simulink model "Vehicle_Model_999_Modular"  (R2025b)
settings: Solver=ode23tb  StartTime=0.0  StopTime=20  MaxStep=0.001  RelTol=1e-3
values from neighbouring files (symbols this model uses):
  aero_par = struct()    [Load_aero_parameters.m]
  init_r = 0    [Run_this_first.m]
  init_vx = 0    [Run_this_first.m]
  init_vy = 0    [Run_this_first.m]
  m = Par.m    [LapSim_Endurance_final_ts_v2.m]    (also in Lap_Sim_Final_inverse.m = Par.Mass; Lapsim_Endurance_final_ts.m; New_LapSim_final_ts_v1.m = Par.Mass; Torque_vectoring_lookup_table_v3.m = 270)
  Par = struct()    [Load_vehicle_parameters.m]
  sus_par = struct()    [Load_sus_parameters.m]
  TireData = []    [Lapsim_final_for_app.m]
  V_ref = 45    [Run_this_first.m]
undefined symbols (not defined in the file or in its folder): Battery, Brake_Val, HP, Ki_data, Kp_data, Motor, steer_input, Steer_Val, Throttle_Val, vx_breakpoints
libraries: simulink x7, autolibshared x2, BatteryEstimators x1, simulink_extras x1
(part 3 of 3)

== matlab function Vehicle_Model_999_Modular/Drivetrain/Thermal/MATLAB Function ==
  settings: updateMethod=DISCRETE  sampleTime=1
  data: Q_total output size=1; I_rms input; Speed_RPM input; P_iron_rotor input; T_motor_K input; T_motor_C output; R_actual output; kt_actual output
function [Q_total, T_motor_C, R_actual, kt_actual] = motor_thermal_logic(I_rms, Speed_RPM, P_iron_rotor, T_motor_K)
    %#codegen
    
    %% 1. Force outputs to be SCALAR doubles
    % This stops the "variable-size matrix" error
    Q_total   = double(0); 
    T_motor_C = double(0);
    R_actual  = double(0);
    kt_actual = double(0);

    %% 2. Constants from Fischer Datasheet
    R_ref   = 0.126;    % Phase resistance at 20°C
    kt_ref  = 0.492;    % Torque constant
    alpha   = 0.00393;  % Temp coefficient for Copper
    gamma_m = 0.001;    % Magnet flux fade (0.1% per degC)
    
    %% 3. Unit Conversion & Calculations
    T_kelvin = double(T_motor_K(1));
    T_motor_C = T_motor_K - 273.15; % Kelvin to Celsius
    
    % Ensure T_motor_C doesn't cause math errors if feedback is zero at start
    R_actual = R_ref * (1 + alpha * (T_motor_C - 20)); 
    kt_actual = kt_ref * (1 - gamma_m * (T_motor_C - 20)); 
    
    % Force I_rms to be treated as a single scalar value
    I_val = double(I_rms(1));
    P_cu = 3 * (I_val^2) * R_actual; 
    
    % Final sum forced to scalar double
    Q_total = P_cu + double(P_iron_rotor(1)); 
end

== matlab function Vehicle_Model_999_Modular/E-powertrain/Motor/Motor with Field Weakening ==
  data: kt input; rpm_4x1 input; Torque_Nm_vec output; throttle_scalar input; v_dc_bus input; Motor parameter; I_dc_total output size=[1]; P_total_sum output size=[1]
function [Torque_Nm_vec, I_dc_total,P_total_sum] = fcn(kt, rpm_4x1, throttle_scalar, v_dc_bus, Motor)
    % Inputs:
    %   rpm_4x1         : [FL; FR; RL; RR] wheel speeds in RPM
    %   throttle_scalar : Driver input (0 to 1)
    %   v_dc_bus        : Battery voltage (V)
    %   Motor           : Struct containing constants
    
    % --- 1. Distribute Inputs ---
    % We apply the same throttle to both motors for now.
    % We extract the Rear-Left (index 3) and Rear-Right (index 4) speeds.
    rpm_targets = [rpm_4x1(3); rpm_4x1(4)]; 
    throttle_vec = [throttle_scalar; throttle_scalar];
    psi_m = kt / (1.5 * Motor.p * sqrt(2)); 

    % Initialize storage
    Torque_Nm_vec = zeros(2, 1); % [T_RL; T_RR]
    P_elec_vec = zeros(2, 1);
    
    for i = 1:2
        % --- 2. Redline & Mechanical Limit Check ---
        if abs(rpm_targets(i)) >= Motor.n_max
            continue; % Torque and Power remain 0
        end

        % --- 3. Electrical Conversions ---
        omega_m = rpm_targets(i) * (2*pi/60);
        omega_e = max(abs(omega_m * Motor.p), 0.1); 
        V_max_phase = v_dc_bus / sqrt(3);
        I_cmd_peak = Motor.I_max_rms * sqrt(2) * throttle_vec(i);

        % --- 4. Region Selection: MTPA vs Field Weakening ---
        V_req_mtpa = omega_e * sqrt((Motor.L * I_cmd_peak)^2 + psi_m^2);
        
        if V_req_mtpa <= V_max_phase
            id = 0;
            iq = I_cmd_peak;
        else
            % Field Weakening logic for Fischer Motor
            a = Motor.L^2;
            b = 2 * Motor.L * psi_m;
            c = Motor.psi_m^2 + (Motor.L * I_cmd_peak)^2 - (V_max_phase / omega_e)^2;
            
            id = (-b + sqrt(max(0, b^2 - 4 * a * c))) / (2 * a);
            id = max(min(id, 0), -I_cmd_peak); 
            iq = sqrt(max(0, I_cmd_peak^2 - id^2));
        end

        % --- 5. Torque and Power Calculation ---
        T_gen = 1.5 * Motor.p * psi_m * iq;
        Torque_Nm_vec(i) = min(T_gen, Motor.T_peak_limit);

        % P_elec = P_mechanical + P_copper_losses
        P_mech = abs(Torque_Nm_vec(i) * omega_m);
        P_copper = 3 * 0.126 * (I_cmd_peak / sqrt(2))^2;
        P_elec_vec(i) = P_mech + P_copper;
    end

    % --- 6. Battery Summation ---
    P_total_sum = sum(P_elec_vec);
    if v_dc_bus > 20
        % Calculate total current draw for the Molicel P45B pack
        I_dc_total = P_total_sum / (0.95 * v_dc_bus);

    else
        I_dc_total = 0;
    end
end

== matlab function Vehicle_Model_999_Modular/Vehicle dynamics/Fx, Fy calculations/Tyre_relaxation/MATLAB Function ==
  data: Fx_ss input; Fx_dot output; Fx_act input; Vx input
function Fx_dot = fcn(Fx_ss, Fx_act, Vx)
    % Fx_ss: Force from Magic Formula block
    % Fx_act: The current integrated force
    % Vx: Longitudinal velocity
    sigma_x = 0.1;
    % Use a small epsilon to avoid division by zero at standstill
    Vx_mod = max(abs(Vx), 0.05); 
    
    % The differential equation
    Fx_dot = (Vx_mod / sigma_x).* (Fx_ss - Fx_act);
end

== matlab function Vehicle_Model_999_Modular/Vehicle dynamics/Fx, Fy calculations/Visualise_Fy_B/MATLAB Function ==
  data: Fy_tire input; Fy_B_fl output; Fy_B_fr output; Fy_B_rl output; Fy_B_rr output
function [Fy_B_fl,Fy_B_fr,Fy_B_rl,Fy_B_rr]  = fcn(Fy_tire)

Fy_B_fl = Fy_tire(1);

Fy_B_fr = Fy_tire(2);

Fy_B_rl = Fy_tire(3);

Fy_B_rr = Fy_tire(4);

end

== matlab function Vehicle_Model_999_Modular/Drivetrain/MATLAB Function ==
  data: T_fl output; T_fr output
function [T_fl,T_fr] = fcn()

T_fl = 0;
T_fr = 0;

== matlab function Vehicle_Model_999_Modular/Vehicle dynamics/Suspension/Camber/DynamicCamber_FromHP_Zmeters ==
  data: Camber output; Zs input; Zs_static input; sus_par parameter; HP parameter; dynamic_camber_visualisation output; static_camber_visualisation output
function [Camber,dynamic_camber_visualisation,static_camber_visualisation] = DynamicCamber_FromHP_Zmeters(Zs,Zs_static,sus_par, HP)
%#codegen
% z_* : wheel vertical displacement (meters, + = bump)
% HP  : hardpoints (mm)
% Output Camber [4x1] radians (dynamic, zeroed at ride height)

% Use this if you have different camber angles for front and rear wheels.
% static_camber_4x1 = [sus_par.Camber_static_f.*ones(2,1) ; ...
                       ...sus_par.Camber_static_r.*ones(2,1)];   
% Assigning values of Zs                           
Zs_1 = Zs(1);
Zs_2 = Zs(2);
Zs_3 = Zs(3);
Zs_4 = Zs(4);
% Assigning values of Zs                           
Zs_1_static = Zs_static(1);
Zs_2_static = Zs_static(2);
Zs_3_static = Zs_static(3);
Zs_4_static = Zs_static(4);
                  
static_camber_4x1 = sus_par.Camber_static.*ones(4,1);

z_FL_static = Zs_1_static * sus_par.Motion_ratio_f;
z_FR_static = Zs_2_static * sus_par.Motion_ratio_f;
z_RL_static = Zs_3_static * sus_par.Motion_ratio_r;
z_RR_static = Zs_4_static * sus_par.Motion_ratio_r;

z_FL = Zs_1 * sus_par.Motion_ratio_f;
z_FR = Zs_2 * sus_par.Motion_ratio_f;
z_RL = Zs_3 * sus_par.Motion_ratio_r;
z_RR = Zs_4 * sus_par.Motion_ratio_r;

%% Convert meters -> mm   (wheel displacement in mm)
zw_FL = z_FL * 1000;
zw_FR = z_FR * 1000;
zw_RL = z_RL * 1000;
zw_RR = z_RR * 1000;

%% Convert meters -> mm   (wheel displacement in mm for _static calculations)
zw_FL_static = z_FL_static * 1000;
zw_FR_static = z_FR_static * 1000;
zw_RL_static = z_RL_static * 1000;
zw_RR_static = z_RR_static * 1000;

%% Absolute camber from geometry

    Camber_FL_d = solveCorner_camber(zw_FL,...
        HP.Front.UCA_F, HP.Front.UCA_R, HP.Front.UCA_O, ...
        HP.Front.LCA_F, HP.Front.LCA_R, HP.Front.LCA_O, ...
        HP.Front.TCP,  1);
    Camber_FL_s = solveCorner_theta(zw_FL_static,...
        HP.Front.UCA_F, HP.Front.UCA_R, HP.Front.UCA_O, ...
        HP.Front.LCA_F, HP.Front.LCA_R, HP.Front.LCA_O, ...
        HP.Front.TCP,  1);

Camber_FL = -Camber_FL_s + Camber_FL_d;

    Camber_FR_d = solveCorner_camber(zw_FR, ...
        HP.Front.UCA_F, HP.Front.UCA_R, HP.Front.UCA_O, ...
        HP.Front.LCA_F, HP.Front.LCA_R, HP.Front.LCA_O, ...
        HP.Front.TCP, -1);
    Camber_FR_s = solveCorner_theta(zw_FR_static, ...
        HP.Front.UCA_F, HP.Front.UCA_R, HP.Front.UCA_O, ...
        HP.Front.LCA_F, HP.Front.LCA_R, HP.Front.LCA_O, ...
        HP.Front.TCP, -1);

Camber_FR = -Camber_FR_d - Camber_FR_s;

    Camber_RL_d =  solveCorner_camber(zw_RL, ...
        HP.Rear.UCA_F, HP.Rear.UCA_R, HP.Rear.UCA_O, ...
        HP.Rear.LCA_F, HP.Rear.LCA_R, HP.Rear.LCA_O, ...
        HP.Rear.TCP,  1);
    Camber_RL_s = solveCorner_theta(zw_RL_static, ...
        HP.Rear.UCA_F, HP.Rear.UCA_R, HP.Rear.UCA_O, ...
        HP.Rear.LCA_F, HP.Rear.LCA_R, HP.Rear.LCA_O, ...
        HP.Rear.TCP,  1);

Camber_RL = Camber_RL_d - Camber_RL_s;

    Camber_RR_d = solveCorner_camber(zw_RR, ...
        HP.Rear.UCA_F, HP.Rear.UCA_R, HP.Rear.UCA_O, ...
        HP.Rear.LCA_F, HP.Rear.LCA_R, HP.Rear.LCA_O, ...
        HP.Rear.TCP, -1);
    Camber_RR_s = solveCorner_theta(zw_RR_static, ...
        HP.Rear.UCA_F, HP.Rear.UCA_R, HP.Rear.UCA_O, ...
        HP.Rear.LCA_F, HP.Rear.LCA_R, HP.Rear.LCA_O, ...
        HP.Rear.TCP, -1);

Camber_RR = -Camber_RR_d - Camber_RR_s;

Camber_abs = [Camber_FL; Camber_FR; Camber_RL; Camber_RR];

%% Dynamic camber (zeroed at ride height)
Camber = Camber_abs + static_camber_4x1;
dynamic_camber_visualisation = [Camber_FL_d;Camber_FR_d;Camber_RL_d;Camber_RR_d];
static_camber_visualisation = [Camber_FL_s;Camber_FR_s;Camber_RL_s;Camber_RR_s];

end

%% Helper function - 1
function Camber = solveCorner_camber(z,UF,UR,UO,LF,LR,LO,TCP,side)
%#codegen
% Returns camber in radians (negative = negative camber)    
%% Mirror for vehicle side
UF(2)=UF(2)*side; UR(2)=UR(2)*side; UO(2)=UO(2)*side;
LF(2)=LF(2)*side; LR(2)=LR(2)*side; LO(2)=LO(2)*side;
TCP(2)=TCP(2)*side;

%% Apply wheel vertical displacement (mm)
UO(3)=UO(3) + z;
LO(3)=LO(3) + z;
TCP(3)=TCP(3) + z;

%% Inner pivots (front view)
UiY = (UF(2)+UR(2))/2;
UiZ = (UF(3)+UR(3))/2;

LiY = (LF(2)+LR(2))/2;
LiZ = (LF(3)+LR(3))/2;

%% Slopes of upper & lower arms
dYU = (UO(2)-UiY);
dYL = (LO(2)-LiY);

if abs(dYU) < 1e-9, dYU = sign(dYU)*1e-9; end
if abs(dYL) < 1e-9, dYL = sign(dYL)*1e-9; end

mU = (UO(3)-UiZ)/dYU;
mL = (LO(3)-LiZ)/dYL;

cU = UiZ - mU*UiY;
cL = LiZ - mL*LiY;

%% Instant Center
den = (mU-mL);
if abs(den) < 1e-9, den = sign(den)*1e-9; end

ICy = (cL-cU)/den;
ICz = mU*ICy + cU;

%% Camber from IC -> Contact Patch (correct definition)
dY = ICy - TCP(2);     % lateral
dZ = ICz - TCP(3);    % vertical

if abs(dZ) < 1e-9, dZ = sign(dZ)*1e-9; end
Camber = -atan(dY/dZ);
end

%% Helper function - 2
function Theta = solveCorner_theta(Z_static,UF,UR,UO,LF,LR,LO,TCP,side)
%% Mirror for vehicle side
    UF(2)=UF(2)*side; UR(2)=UR(2)*side; UO(2)=UO(2)*side;
    LF(2)=LF(2)*side; LR(2)=LR(2)*side; LO(2)=LO(2)*side;
    TCP(2)=TCP(2)*side;
    
    %% Apply wheel vertical displacement (mm)
    UO(3)=UO(3) + Z_static;
    LO(3)=LO(3) + Z_static;
    TCP(3)=TCP(3) + Z_static;
    
    %% Inner pivots (front view)
    UiY = (UF(2)+UR(2))/2;
    UiZ = (UF(3)+UR(3))/2;
    
    LiY = (LF(2)+LR(2))/2;
    LiZ = (LF(3)+LR(3))/2;
    
    %% Slopes of upper & lower arms
    dYU = (UO(2)-UiY);
    dYL = (LO(2)-LiY);
    
    if abs(dYU) < 1e-9, dYU = sign(dYU)*1e-9; end
    if abs(dYL) < 1e-9, dYL = sign(dYL)*1e-9; end
    
    mU = (UO(3)-UiZ)/dYU;
    mL = (LO(3)-LiZ)/dYL;
    
    cU = UiZ - mU*UiY;
    cL = LiZ - mL*LiY;
    
    %% Instant Center
    den = (mU-mL);
    if abs(den) < 1e-9, den = sign(den)*1e-9; end
    
    ICy = (cL-cU)/den;
    ICz = mU*ICy + cU;
    
    %% Camber from IC -> Contact Patch (correct definition)
    dY = ICy - TCP(2);     % lateral
    dZ = ICz - TCP(3);    % vertical
    
    if abs(dZ) < 1e-9, dZ = sign(dZ)*1e-9; end
    
    Theta = abs(atan(dY/dZ));
end

== matlab function Vehicle_Model_999_Modular/Vehicle dynamics/Suspension/Normal_loads1/ARB/MATLAB Function ==
  data: Zs input; F_arb output; sus_par parameter
function F_arb = fcn(Zs,sus_par)

  % Calculation of Anti roll bar forces at each wheel
    delta_zf = Zs(1) - Zs(2);
    delta_zr = Zs(3) - Zs(4);

    F_arb_fl = sus_par.K_arb_f*delta_zf/2;
    F_arb_fr = -sus_par.K_arb_f*delta_zf/2;
    F_arb_rl = sus_par.K_arb_r*delta_zr/2;
    F_arb_rr = -sus_par.K_arb_r*delta_zr/2;

    F_arb = [F_arb_fl ; F_arb_fr ; F_arb_rl ; F_arb_rr];

== matlab function Vehicle_Model_999_Modular/Vehicle dynamics/Suspension/Normal_loads1/MATLAB Function ==
  data: F_arb input; F_spring input; Fz output; Par parameter
function Fz = fcn(F_arb , F_spring,Par)
m_us = [12;12;18;18];
g = Par.g;
F_unsprung = m_us.*g;
Fz = F_unsprung - (F_spring + F_arb);

== matlab function Vehicle_Model_999_Modular/Vehicle dynamics/Suspension/Normal_loads1/Spring_forces/MATLAB Function ==
  data: theta input; phi input; F_aero_total input; Zs output size=[4 1]; F_spring output; Par parameter; aero_par parameter; sus_par parameter; TireData parameter; Zs1 output size=[4 1]
function [Zs,F_spring,Zs1] = fcn(theta, phi, F_aero_total, Par, aero_par, sus_par,TireData)

  % 1. Constants
    g = Par.g;
    Lf = Par.Lf;  % Front wheel base
    Lr = Par.Lr;  % Rear wheel base
    T = Par.TW;
    ms = Par.sprung_mass;
    half_T = T/2;
   

    % Calculating Pitching stiffness
    Kw_fl = sus_par.Ks_f.*(sus_par.Motion_ratio_f)^2; 
    Kw_fr = sus_par.Ks_f.*(sus_par.Motion_ratio_f)^2;
    Kw_rl = sus_par.Ks_r.*(sus_par.Motion_ratio_r)^2;
    Kw_rr = sus_par.Ks_r.*(sus_par.Motion_ratio_r)^2;

    Kw = [Kw_fl;Kw_fr;Kw_rl;Kw_rr];

    % Static load due to sprung mass and unsprung mass at each wheel
    F_sprung_mass = ms*g/4;
    % Stiffness at each wheel:
    Kt = TireData.VERTICAL_STIFFNESS;
    stiff_1 = Kw(1) * Kt /(Kw(1) + Kt);
    stiff_2 = Kw(2) * Kt /(Kw(2) + Kt);
    stiff_3 = Kw(3) * Kt /(Kw(3) + Kt);
    stiff_4 = Kw(4) * Kt /(Kw(4) + Kt);
    
    % Vertical deflection of each suspension(compression = -ve)
    zsfl = -(F_sprung_mass)/stiff_1 + Lf*theta + (half_T)*phi - 0.5 * F_aero_total * (1 - aero_par.CP_rear)/stiff_1;
    zsfr = -(F_sprung_mass)/stiff_2 + Lf*theta - (half_T)*phi - 0.5 * F_aero_total * (1 - aero_par.CP_rear)/stiff_2;
    zsrl = -(F_sprung_mass)/stiff_3 - Lr*theta + (half_T)*phi - 0.5 * F_aero_total*(aero_par.CP_rear)/stiff_3;
    zsrr = -(F_sprung_mass)/stiff_4 - Lr*theta - (half_T)*phi - 0.5 * F_aero_total*(aero_par.CP_rear)/stiff_4;

    Zs = [zsfl;zsfr;zsrl;zsrr];


      % Vertical deflection of each suspension(compression = -ve) for ...
      ...camber calculations
    zsfl_1 = -(F_sprung_mass)/stiff_1 ;
    zsfr_1 = -(F_sprung_mass)/stiff_2 ;
    zsrl_1 = -(F_sprung_mass)/stiff_3 ;
    zsrr_1 = -(F_sprung_mass)/stiff_4 ;

    Zs1 = [zsfl_1;zsfr_1;zsrl_1;zsrr_1];

    % Spring force at each wheel
    Fs_fl = stiff_1*zsfl;
    Fs_fr = stiff_2*zsfr;
    Fs_rl = stiff_3*zsrl;
    Fs_rr = stiff_4*zsrr;

    F_spring = [Fs_fl;Fs_fr;Fs_rl;Fs_rr];

== matlab function Vehicle_Model_999_Modular/Vehicle dynamics/Suspension/Normal_loads1/Visualise sus disp/Zs in mm ==
  data: Zs input; zsfl output; zsfr output; zsrl output; zsrr output
function [zsfl,zsfr,zsrl,zsrr] = fcn(Zs)

zsfl = Zs(1);
zsfr = Zs(2);
zsrl = Zs(3);
zsrr = Zs(4);

end

== matlab function Vehicle_Model_999_Modular/Vehicle dynamics/Suspension/roll and pitch angles1/Phi_constants ==
  data: K_phi output; C_phi output; Par parameter; sus_par parameter
function [K_phi,C_phi] = fcn(Par, sus_par)

% Calculating Pitching stiffness
Kw_fl = sus_par.Ks_f.*(sus_par.Motion_ratio_f)^2; 
Kw_fr = sus_par.Ks_f.*(sus_par.Motion_ratio_f)^2;
Kw_rl = sus_par.Ks_r.*(sus_par.Motion_ratio_r)^2;
Kw_rr = sus_par.Ks_r.*(sus_par.Motion_ratio_r)^2;

K_phi = (Kw_fl + Kw_fr).*(Par.TW/2)^2 + (Kw_rl + Kw_rr).*(Par.TW/2)^2;

% Calculating Pitch Damping
Cw_fl = sus_par.C_damp_f.*(sus_par.Motion_ratio_f)^2;
Cw_fr = sus_par.C_damp_f.*(sus_par.Motion_ratio_f)^2;
Cw_rl = sus_par.C_damp_r.*(sus_par.Motion_ratio_r)^2;
Cw_rr = sus_par.C_damp_r.*(sus_par.Motion_ratio_r)^2;

C_phi = (Cw_fl + Cw_fr).*(Par.TW/2)^2 + (Cw_rl + Cw_rr).*(Par.TW/2)^2;

== matlab function Vehicle_Model_999_Modular/Vehicle dynamics/Suspension/roll and pitch angles1/theta_constants ==
  data: K_theta output; C_theta output; sus_par parameter; Par parameter
function [K_theta,C_theta] = fcn(sus_par,Par)

% Calculating Pitching stiffness
Kw_fl = sus_par.Ks_f.*(sus_par.Motion_ratio_f)^2; 
Kw_fr = sus_par.Ks_f.*(sus_par.Motion_ratio_f)^2;
Kw_rl = sus_par.Ks_r.*(sus_par.Motion_ratio_r)^2;
Kw_rr = sus_par.Ks_r.*(sus_par.Motion_ratio_r)^2;

K_theta = (Kw_fl + Kw_fr).*(Par.Lf)^2 + (Kw_rl + Kw_rr).*(Par.Lr)^2;

% Calculating Pitch Damping
Cw_fl = sus_par.C_damp_f.*(sus_par.Motion_ratio_f)^2;
Cw_fr = sus_par.C_damp_f.*(sus_par.Motion_ratio_f)^2;
Cw_rl = sus_par.C_damp_r.*(sus_par.Motion_ratio_r)^2;
Cw_rr = sus_par.C_damp_r.*(sus_par.Motion_ratio_r)^2;

C_theta = (Cw_fl + Cw_fr).*(Par.Lf)^2 + (Cw_rl + Cw_rr).*(Par.Lr)^2;

% Kw = [Kw_fl;Kw_fr;Kw_rl;Kw_rr];

== matlab function Vehicle_Model_999_Modular/E-powertrain/Motor/rpm selection for third wheel ==
  data: u input; y output
function y = fcn(u)

y = u(3);

== matlab function Vehicle_Model_999_Modular/Vehicle dynamics/Fx, Fy calculations/Slip_angle_calculation/Slip Angles ==
  data: Longitudinal_vel input; slip_angles output; Lateral_vel input; yawrate input; Steer_FL input; Steer_FR input; Par parameter
function slip_angles = fcn(Longitudinal_vel, Lateral_vel, yawrate, Steer_FL, Steer_FR, Par)
%#codegen

    % 1. Geometry Setup
    L = Par.WB;
    T = Par.TW;
    
    % Distance from CG to Axles
    a = L * Par.WD_r;     
    b = L - a;             
    half_T = T / 2;

    % 2. Calculate Velocity Components at Each Corner
    % Kinematic transformation from CG to Hubs
    % Front Left (1)
        Vx_FL = Longitudinal_vel - yawrate * half_T;
        Vy_FL = Lateral_vel + yawrate * a;
    
    % Front Right (2)
        Vx_FR = Longitudinal_vel + yawrate * half_T;
        Vy_FR = Lateral_vel + yawrate * a;
    
    % Rear Left (3)
        Vx_RL = Longitudinal_vel - yawrate * half_T;
        Vy_RL = Lateral_vel - yawrate * b;
    
    % Rear Right (4)
        Vx_RR = Longitudinal_vel + yawrate * half_T;
        Vy_RR = Lateral_vel - yawrate * b;

    % 3. Calculate Velocity Angles (Theta_V)

        Theta_FL = atan2(Vy_FL, max(Vx_FL,0.01)); 
        Theta_FR = atan2(Vy_FR, max(Vx_FR,0.01));
        Theta_RL = atan2(Vy_RL, max(Vx_RL,0.01));
        Theta_RR = atan2(Vy_RR, max(Vx_RR,0.01));
    
    % 4. Construct Steering Vector (Delta)
    % Rears are assumed fixed (0 steering)
        Delta = [Steer_FL; Steer_FR; 0; 0];
    
    % Vector of Velocity Angles
        Theta_V = [Theta_FL; Theta_FR; Theta_RL; Theta_RR];

    % 5. Final Calculation
    % Alpha = Delta - Theta_V
        slip_angles = Delta - Theta_V ;
end

== matlab function Vehicle_Model_999_Modular/Vehicle dynamics/Fx, Fy calculations/Slip_ratio_calculation/slip ratios ==
  data: Vx input; Vy input; slip_ratios output; yawrate input; Omega input; Steer_FL input; Steer_FR input; Par parameter
function slip_ratios = fcn(Vx,Vy, yawrate, Omega,Steer_FL,Steer_FR, Par)
%#codegen


    % 1. Constants
    T = Par.TW;
    Re = Par.R0;
    half_T = T / 2;
    a= Par.Lf;
    b=Par.Lr;
    r = yawrate;
    % 2 Yaw Rate Correction (Kinematics)
    
    Vx_FL = Vx - yawrate * half_T;  % Left
    Vx_FR = Vx + yawrate * half_T;  % Right
    Vx_RL = Vx - yawrate * half_T;
    Vx_RR = Vx + yawrate * half_T;
    
    Vx_vec = [Vx_FL; Vx_FR; Vx_RL; Vx_RR];
    
    Vy_FL = Vy + r * a;
    Vy_FR = Vy+ r * a;
    Vy_RL = Vy- r * b;
    Vy_RR = Vy- r * b;

    Vy_vec = [Vy_FL; Vy_FR; Vy_RL; Vy_RR];
    Delta = [Steer_FL;Steer_FR;0;0];
    % 3. Slip Angle Correction (Projection)
 
    V_road_plane = Vx_vec .* cos(Delta) + Vy_vec .* sin(Delta);

    % 4. Calculate Wheel Linear Speed
    V_wheel = Omega .* Re;

    % 5. Calculate Slip Ratio
    V_safe_threshold = 0.1; 
    V_ref = max(abs(V_road_plane), V_safe_threshold);
    
    slip_ratios_raw = (V_wheel - V_road_plane) ./ V_ref;
    slip_ratios = slip_ratios_raw;
    % slip_ratios = min(max(slip_ratios_raw,-1),1);
end

== matlab function Vehicle_Model_999_Modular/Vehicle dynamics/Steering/Steering Kinematics/Steering Kinematics ==
  data: Steer_Input input; Ackermann_Pct input; Steer_FL output; Steer_FR output; Par parameter
function [Steer_FL, Steer_FR] = fcn(Steer_Input, Ackermann_Pct, Par)
%#codegen

    % 1. Constants
    L = Par.WB;      % Wheelbase
    half_T = Par.TW / 2; % Half Track Width

    % 2. Safety Clamp (Prevent tan(90) singularity)
    delta = min(max(Steer_Input, -1.5), 1.5); 
    
    % 3. Calculate "Pure Ackermann" Angles
    % Ideally, inner wheel turns sharper than outer wheel.
    tan_d = tan(delta);
    
    % FL (Left): Denom depends on sign of turn.
    % If turning Left (+), Denom shrinks (Sharper).
    FL_Ack = atan( (L * tan_d) / (L - half_T * tan_d) );
    
    % FR (Right): 
    % If turning Left (+), Denom grows (Shallower).
    FR_Ack = atan( (L * tan_d) / (L + half_T * tan_d) );
    
    % 4. Calculate "Parallel" Angles
    % Both wheels exactly match the center input
    FL_Par = delta;
    FR_Par = delta;
    
    % 5. Linear Blend based on Percentage
    % Formula: Final = Parallel + (Ackermann - Parallel) * Percent
    Steer_FL = FL_Par + (FL_Ack - FL_Par) * Ackermann_Pct;
    Steer_FR = FR_Par + (FR_Ack - FR_Par) * Ackermann_Pct;

end

== matlab function Vehicle_Model_999_Modular/Vehicle dynamics/Fx, Fy calculations/Simplified Tire Model ==
  data: Fz input; Fx output size=4; slip_ratios input; slip_angles input; camber_angles input; Fy output size=4; Self_aligning_torque output size=4; Mu_x output size=4; Mu_y output size=4; TireData parameter; Par parameter; sus_par parameter; Dy output size=[4 1]
function [Fx, Fy, Self_aligning_torque, Mu_x, Mu_y, Dy] = fcn(Fz, slip_ratios, slip_angles, camber_angles, TireData, Par, sus_par)
%#codegen
% =========================================================================
%  VECTORIZED MAGIC FORMULA 5.2 (4-WHEEL)
% =========================================================================

    % 0. Enforce Column Vectors (Crash Protection)
    Fz = Fz(:);
    slip_ratios = slip_ratios(:);
    slip_angles = slip_angles(:);
    camber_angles = camber_angles(:);

    % 1. EXTRACT PARAMETERS (Scalars)
    p = TireData;
    s = TireData.Scales;
    Fz0 = p.FNOMIN;
    R0  = p.R0;
    par = Par;
    
    % 2. INPUT SAFETY & NORMALIZATION
    % Clamp negative loads to 0 (Tires can't pull ground)
    Fz_safe = max(Fz, 0); 
    
    % Avoid division by zero for Mu calculations later
    Fz_denom = max(Fz_safe, 1.0); 
    
    % Normalized Load (dfz) - Vectorized
    dfz = (Fz_safe - Fz0) ./ Fz0;
    
    % ---------------------------------------------------------------------
    % A. LONGITUDINAL FORCE (Fx) - VECTORIZED
    % ---------------------------------------------------------------------
    Cx = p.PCX1 * s.LCX;
    
    % Friction Coeff Mu_x
    mu_x_base = (p.PDX1 + p.PDX2 .* dfz) .* (1 - p.PDX3 .* camber_angles.^2) .* s.LMUX;
    Dx = mu_x_base .* Fz_safe;
    
    % Stiffness Kx
    Kx = Fz_safe .* (p.PKX1 + p.PKX2 .* dfz) .* exp(p.PKX3 .* dfz) .* s.LKX;
    
    % Stiffness Factor Bx
    Bx = Kx ./ (Cx .* Dx + 1e-6); 
    
    % Shifts (Horizontal & Vertical)
    Shx = (p.PHX1 + p.PHX2 .* dfz) .* s.LHX;
    Svx = Fz_safe .* (p.PVX1 + p.PVX2 .* dfz) .* s.LVX;
    
    % Composite Slip
    k_s = slip_ratios + Shx;
    
    % Curvature Ex (Sign Dependent)
    Ex = (p.PEX1 + p.PEX2 .* dfz + p.PEX3 .* dfz.^2) .* (1 - p.PEX4 .* sign(k_s)) .* s.LEX;
    Ex(Ex > 1) = 1; % Clamp
    
    % Calculation
    Bx_k = Bx .* k_s;
    Fx = Dx .* sin(Cx .* atan(Bx_k - Ex .* (Bx_k - atan(Bx_k)))) + Svx;
    
    % ---------------------------------------------------------------------
    % B. LATERAL FORCE (Fy) - VECTORIZED
    % ---------------------------------------------------------------------
    Cy = p.PCY1 * s.LCY;
    
    % Friction Coeff Mu_y
    mu_y_base = (p.PDY1 + p.PDY2 .* dfz) .* (1 - p.PDY3 .* camber_angles.^2) .* s.LMUY;
    Dy = mu_y_base .* Fz_safe;
    
    % Cornering Stiffness Ky (Trig Form)
    Ky = p.PKY1 .* Fz0 .* sin(2 .* atan(Fz_safe ./ (p.PKY2 .* Fz0))) .* (1 - p.PKY3 .* abs(camber_angles)) .* s.LKY;
    
    % Poly fallback check (if PKY2 implies poly form)
    if (Ky(1) < 1)
        Ky = Fz_safe .* (p.PKY1 + p.PKY2 .* dfz) .* s.LKY;
    end
    
    By = Ky ./ (Cy .* Dy + 1e-6);
    
    % Shifts 
    Shy = (p.PHY1 + p.PHY2 .* dfz) .* s.LHY;
    Svy = Fz_safe .* (p.PVY1 + p.PVY2 .* dfz) .* s.LVY;
    
    % FIXED: Removed the 0* debug multiplier
    a_s = slip_angles + Shy;
    
    % Curvature Ey (Sign Dependent)
    Ey = (p.PEY1 + p.PEY2 .* dfz) .* (1 - (p.PEY3 + p.PEY4 .* camber_angles) .* sign(a_s)) .* s.LEY;
    Ey(Ey > 1) = 1;
    
    % Calculation
    By_a = By .* a_s;
    % FIXED: Removed the 0* debug multiplier
    Fy = -(Dy .* sin(Cy .* atan(By_a - Ey .* (By_a - atan(By_a)))) + Svy);
    
    % ---------------------------------------------------------------------
    % C. SELF-ALIGNING TORQUE (Mz) - VECTORIZED
    % ---------------------------------------------------------------------
    % Peak Trail Dt
    Dt = (p.QDZ1 + p.QDZ2 .* dfz) .* (1 - p.QDZ3 .* abs(camber_angles)) .* R0 .* s.LTR;
    
    % Trail Slope Bt
    Bt = (p.QBZ1 + p.QBZ2 .* dfz + p.QBZ3 .* dfz.^2) .* (1 + p.QBZ4 .* abs(camber_angles)) .* (s.LKY / s.LMUY);
    
    Ct = p.QCZ1; % Scalar
    Et = (p.QEZ1 + p.QEZ2 .* dfz + p.QEZ3 .* dfz.^2);
    
    % Trail 't' Calculation(Pneumatic trail)
    Bt_a = Bt .* a_s;
    alpha_t = Bt_a - Et .* (Bt_a - atan(Bt_a));
    t = Dt .* cos(Ct .* atan(alpha_t)) .* cos(a_s);
    
    % Trail 'tm' Calculation(mechanical trail)
    tm = par.R0 .* tan(sus_par.Caster_static);
    
    % Residual Mzr
    Dr = Fz_safe .* R0 .* (p.QDZ6 + p.QDZ7 .* dfz) .* s.LRES;
    Br = 10;
    Mzr = Dr .* cos(atan(Br .* a_s));
    
    % Final Mz (Standard Restoring: Negative Slope)
    Self_aligning_torque = -(t + tm) .* Fy + Mzr;
    
    % ---------------------------------------------------------------------
    % D. OUTPUTS 
    % ---------------------------------------------------------------------
    % Friction Coeffs
    Mu_x = Fx ./ Fz_denom;
    Mu_y = Fy ./ Fz_denom;
    
    % Note on Lifted Wheels: Because Fz_safe mathematically zeroes out 
    % Dx, Kx, Dy, Ky, Dt, and Dr, the outputs smoothly evaluate to 0 
    % without needing the commented-out boolean masking. 
    % This is faster and safer for C-code generation.
end
